simulink model "ADAS_System"  (R2025b)
settings: Solver=VariableStepAuto  StartTime=0.0  StopTime=10.0  RelTol=1e-3
values from neighbouring files (symbols this model uses):
  fs = 100    [fuzzy_in_workspace.mat]    (also in init_ADAS.m)
  v_lead = 20    [fuzzy_in_workspace.mat]    (also in init_ADAS.m = 0)
libraries: simulink x2
settings Model: Creator=szymo  LastModifiedBy=firiusz

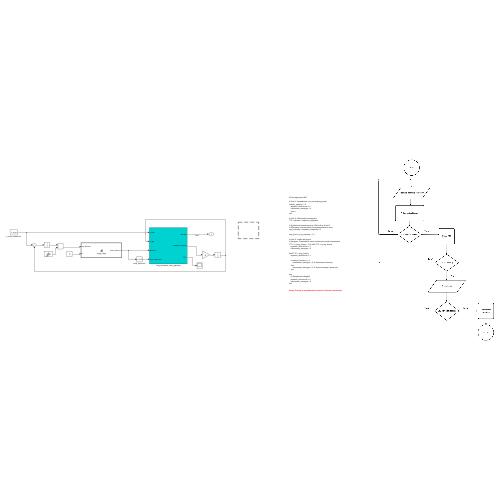
[thumbnail: Simulink's stored preview of the top-level diagram]
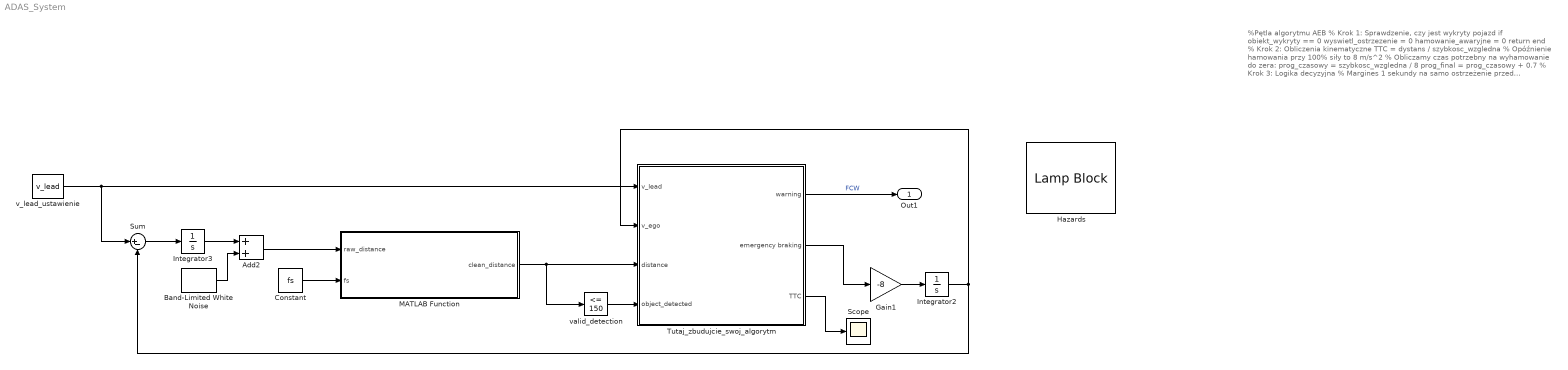
== system ADAS_System ==
  note: %Pętla algorytmu AEB
      |
      | % Krok 1: Sprawdzenie, czy jest wykryty pojazd
      | if obiekt_wykryty == 0
      | wyswietl_ostrzezenie = 0
      | hamowanie_awaryjne = 0
      | return
      | end
      |
      | % Krok 2: Obliczenia kinematyczne
      | TTC = dystans / szybkosc_wzgledna
      |
      | % Opóźnienie hamowania przy 100% siły to 8 m/s^2
      | % Obliczamy czas potrzebny na wyhamowanie do zera:
      | prog_czasowy = szybkosc_wzgledna / 8
      |
      | prog_final = prog_czasowy + 0.7
      |
      | % Krok 3: Logika decyzyjna
      | % Margines 1 sekundy na samo ostrzeżenie przed hamowaniem
      | if TTC < (prog_finalny + 1.0) AND TTC >= prog_finalny
      | wyswietl_ostrzezenie = 1
      | hamowanie_awaryjne = 0
      |
      | elseif TTC < prog_finalny
      | wyswietl_ostrzezenie = 1
      |
      | if reakcja_kierowcy == 1
      | hamowanie_awaryjne = 0 % Hamowanie kierowcy
      | else
      | hamowanie_awaryjne = 1 % System hamuje z pełną siłą
      | end
      |
      | else
      | % Bezpieczna odległość
      | wyswietl_ostrzezenie = 0
      | hamowanie_awaryjne = 0
      | end
      |
      | Uwagi: Zmiany w pseudokodzie oznaczać kolorem czerwonym
  Add2 : Sum
  Band-Limited White Noise : simulink/Sources/Band-Limited White Noise  Cov=[0.1]  Ts=0.1  seed=[23341]
  Constant : Constant  Value=fs
  Gain1 : Gain  Gain=-8
  Hazards : LampBlock  LabelPosition=Bottom  DefaultColor=[192.0, 192.0, 192.0]  Icon=Hazards
  Integrator2 : Integrator  InitialCondition=30
  Integrator3 : Integrator  InitialCondition=200
  MATLAB Function : MATLAB Function  TreatAsAtomicUnit=on
  Scope : Scope
      settings: ActiveDisplayYMinimum=25.38133581091526  ActiveDisplayYMaximum=43.98552342851103
  Sum : Sum  Inputs=|+-
  Tutaj_zbudujcie_swoj_algorytm : Subsystem
  v_lead_ustawienie : Constant  Value=v_lead
  valid_detection : simulink/Logic and Bit Operations/Compare To Constant  relop=<=  const=150  OutDataTypeStr=boolean
  Out1 : Outport
  wires:
  Band-Limited White Noise/1 -> Add2/2
  Add2/1 -> MATLAB Function/1(raw_distance)
  Constant/1 -> MATLAB Function/2(fs)
  Tutaj_zbudujcie_swoj_algorytm/2(emergency braking) -> Gain1/1
  Gain1/1 -> Integrator2/1
  Integrator2/1 -> Tutaj_zbudujcie_swoj_algorytm/2(v_ego), Sum/2
  v_lead_ustawienie/1 -> Sum/1, Tutaj_zbudujcie_swoj_algorytm/1(v_lead)
  Sum/1 -> Integrator3/1
  Integrator3/1 -> Add2/1
  MATLAB Function/1(clean_distance) -> valid_detection/1, Tutaj_zbudujcie_swoj_algorytm/3(distance)
  valid_detection/1 -> Tutaj_zbudujcie_swoj_algorytm/4(object_detected)
  Tutaj_zbudujcie_swoj_algorytm/1(warning) -> Out1/1  "FCW"
  Tutaj_zbudujcie_swoj_algorytm/3("TTC ") -> Scope/1

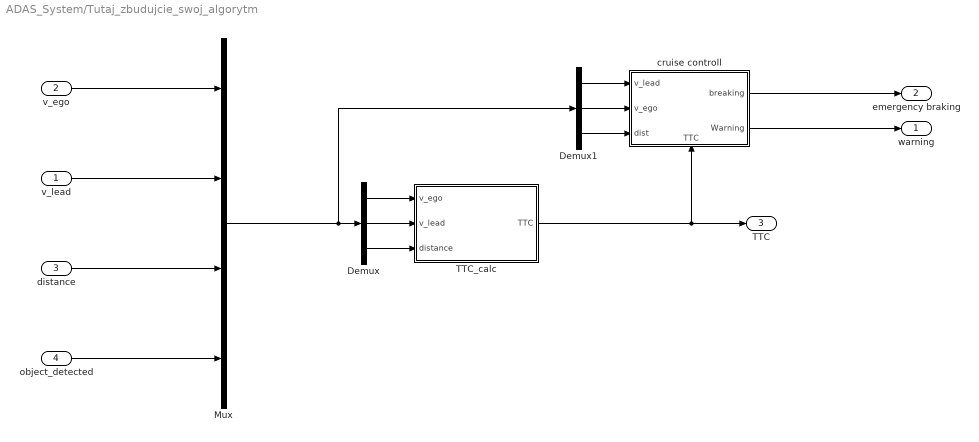
== system ADAS_System/Tutaj_zbudujcie_swoj_algorytm ==
  v_lead : Inport
  v_ego : Inport  Port=2
  distance : Inport  Port=3
  object_detected : Inport  Port=4
  Demux : Demux  Outputs=3
  Demux1 : Demux  Outputs=3
  Mux : Mux
  TTC_calc : Subsystem
  cruise controll : Subsystem
      settings: PortSchema="{\"entries\":[{\"content\":{\"sides\":[{\"content\":{\"connectorIds\":[\"In1\",\"In2\",\"In3\"]},\"type\":\"ConnectorPlacement.EquallySpacedRectSide\",\"uuid\":\"b29f8bd9-5ab8-4e5a-bf6b-e5a68341bc73\"},{\"content\":{\"connectorIds\":[\"Out1\",\"Out2\"],\"side\":\"RIGHT\"},\"type\":\"ConnectorPlacement.EquallySpacedRectSide\",\"uuid\":\"9c58c752-7d1a-430a-8670-77f51b475624\"},{\"content\":{\"side\":\"TOP\"},\"type\":\"ConnectorPlacement.EquallySpacedRectSide\",\"uuid\":\"c2a3ee0e-6e0d-48d5-95c7-ab1f30ef8b3c\"},{\"content\":{\"connectorIds\":[\"In4\"],\"side\":\"BOTTOM\"},\"type\":\"ConnectorPlacement.EquallySpacedRectSide\",\"uuid\":\"2c174705-14d9-4020-a391-f7a929ebd812\"}]},\"type\":\"ConnectorPlacement.EquallySpacedConnector\",\"uuid\":\"89e3bd94-99d2-454b-91a5-f54c08e29716\"}],\"packageUris\":[\"http://schema.mathworks.com/mf0/Connector/R2020b\"],\"version\":\"1.0\"}"
  warning : Outport
  emergency braking : Outport  Port=2
  "TTC " : Outport  Port=3
  wires:
  TTC_calc/1(TTC) -> cruise controll/4(TTC), "TTC "/1
  v_ego/1 -> Mux/1
  v_lead/1 -> Mux/2
  distance/1 -> Mux/3
  object_detected/1 -> Mux/4
  Demux/1 -> TTC_calc/1(v_ego)
  Demux/2 -> TTC_calc/2(v_lead)
  Demux/3 -> TTC_calc/3(distance)
  Mux/1 -> Demux1/1, Demux/1
  Demux1/1 -> cruise controll/1(v_lead)
  Demux1/2 -> cruise controll/2(v_ego)
  Demux1/3 -> cruise controll/3(dist)
  cruise controll/1(breaking) -> emergency braking/1
  cruise controll/2(Warning) -> warning/1

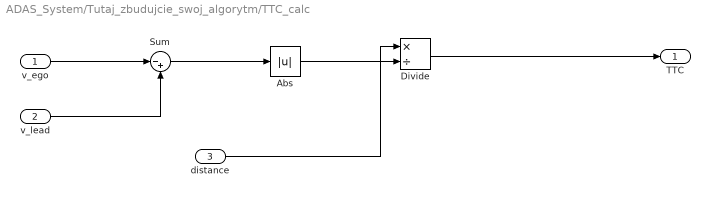
== system ADAS_System/Tutaj_zbudujcie_swoj_algorytm/TTC_calc ==
  v_ego : Inport
  v_lead : Inport  Port=2
  distance : Inport  Port=3
  Abs : Abs  SaturateOnIntegerOverflow=off
  Divide : Product  Inputs=*/
  Sum : Sum  Inputs=|-+
  TTC : Outport
  wires:
  Divide/1 -> TTC/1
  v_lead/1 -> Sum/2
  v_ego/1 -> Sum/1
  distance/1 -> Divide/1
  Sum/1 -> Abs/1
  Abs/1 -> Divide/2

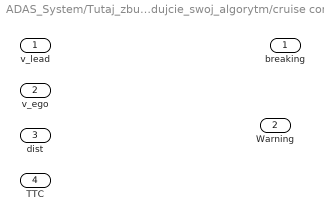
== system ADAS_System/Tutaj_zbudujcie_swoj_algorytm/cruise controll ==
  v_lead : Inport
  v_ego : Inport  Port=2
  dist : Inport  Port=3
  TTC : Inport  Port=4
  breaking : Outport
  Warning : Outport  Port=2

== matlab function ADAS_System/MATLAB Function ==
  settings: updateMethod=DISCRETE
  data: raw_distance input; clean_distance output; fs input
function clean_distance = radar_filter(raw_distance, fs)
    persistent last_dist;
    
    % Inicjalizacja przy pierwszym kroku symulacji
    if isempty(last_dist)
        last_dist = raw_distance;
    end  
    
    % Obliczenie kroku czasu na podstawie częstotliwości próbkowania
    dt = 1 / fs; 
    
    tau = 0.02; 
    
    % Dynamiczne obliczenie wagi dla nowego pomiaru
    alpha = dt / (tau + dt); 
    
    % Filtracja: waga_nowego * nowy_pomiar + waga_starego * stary_pomiar
    clean_distance = alpha * raw_distance + (1 - alpha) * last_dist;
    
    % Zapisanie obecnej wartości na potrzeby kolejnego kroku
    last_dist = clean_distance;
end
